simulink model "GettingStarted"  (R2015b)
settings: Solver=VariableStepAuto  StartTime=0.0  StopTime=inf  RelTol=1e-3
settings Model: Creator=mihai.ciobanu  LastModifiedBy=mihai.ciobanu

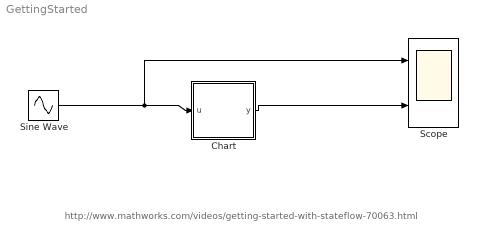
== system GettingStarted ==
  note: http://www.mathworks.com/videos/getting-started-with-stateflow-70063.html
  Chart : Stateflow chart  TreatAsAtomicUnit=on
  Scope : Scope  NumInputPorts=2
  Sine Wave : Sin  SampleTime=0
  wires:
  Sine Wave/1 -> Scope/1, Chart/1(u)
  Chart/1(y) -> Scope/2

== stateflow chart GettingStarted/Chart ==
  state ON
    entry: y=1;
  state OFF
    entry: y=-1;
  (default) -> ON
  ON -> OFF : [u>0]
  OFF -> ON : [u<0]
  data: u input; y output
